simulink model "lab4_3_"  (R2023b)
settings: Solver=VariableStepAuto  StartTime=0.0  StopTime=50  RelTol=1e-3
settings Model: Creator=diontep  LastModifiedBy=lizar

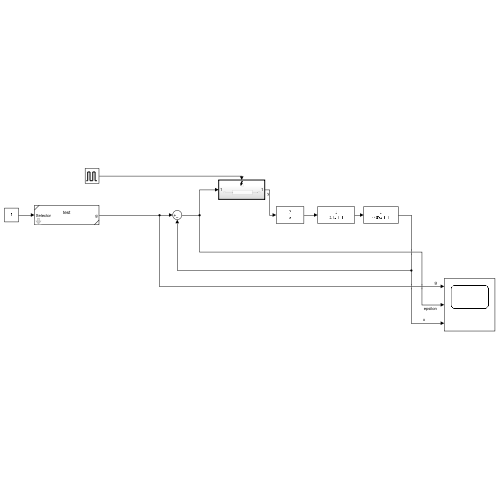
[thumbnail: Simulink's stored preview of the top-level diagram]
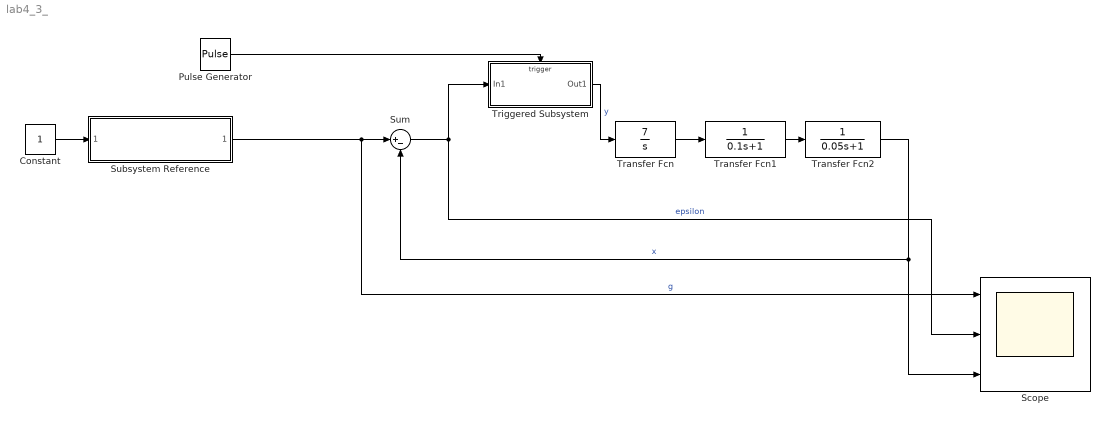
== system lab4_3_ ==
  Constant : Constant
  Pulse Generator : DiscretePulseGenerator  PulseType=Time based  Period=0.01  PulseWidth=50
  Scope : Scope  NumInputPorts=3
  Subsystem Reference : Subsystem  ReferencedSubsystem=test  k1=1  k2=50  k3=100
  Sum : Sum  Inputs=|+-
  Transfer Fcn : TransferFcn  Numerator=[7]  Denominator=[1 0]
  Transfer Fcn1 : TransferFcn  Denominator=[0.1 1]
  Transfer Fcn2 : TransferFcn  Denominator=[0.05 1]
  Triggered Subsystem : Subsystem  TreatAsAtomicUnit=on
  wires:
  Sum/1 -> Triggered Subsystem/1(In1), Scope/2  "epsilon"
  Transfer Fcn/1 -> Transfer Fcn1/1
  Transfer Fcn1/1 -> Transfer Fcn2/1
  Transfer Fcn2/1 -> Sum/2, Scope/3  "x"
  Pulse Generator/1 -> Triggered Subsystem/Trigger
  Subsystem Reference/1 -> Scope/1, Sum/1  "g"
  Triggered Subsystem/1(Out1) -> Transfer Fcn/1  "y"
  Constant/1 -> Subsystem Reference/1

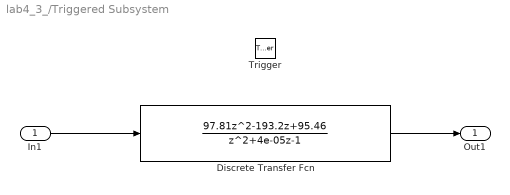
== system lab4_3_/Triggered Subsystem ==
  In1 : Inport
  Trigger : TriggerPort  VariantControl=(inherit)
  Discrete Transfer Fcn : DiscreteTransferFcn  Numerator=[97.81 -193.2 95.46]  Denominator=[1 4e-05 -1]
  Out1 : Outport
  wires:
  In1/1 -> Discrete Transfer Fcn/1
  Discrete Transfer Fcn/1 -> Out1/1
